simulink model "simulink_projekt3"  (R2023b)
settings: Solver=VariableStepAuto  StartTime=0.0  StopTime=5  RelTol=1e-3
settings Model: Creator=ingrj  LastModifiedBy=ingrj

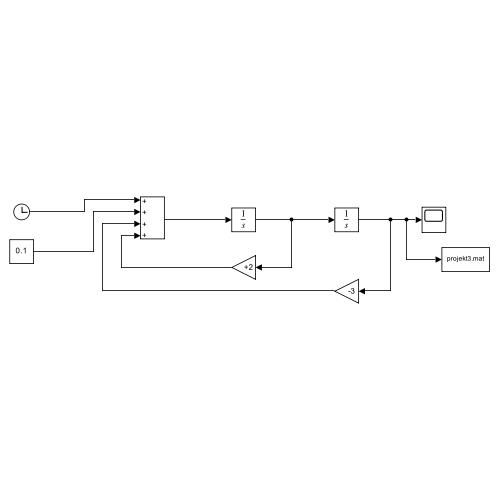
[thumbnail: Simulink's stored preview of the top-level diagram]
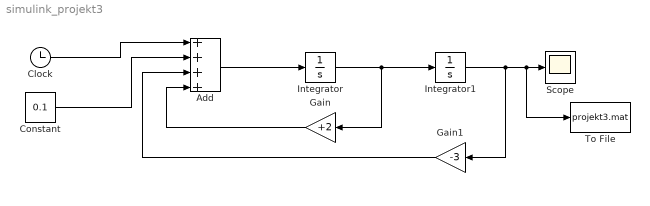
== system simulink_projekt3 ==
  Add : Sum  Inputs=++++
  Clock : Clock
  Constant : Constant  Value=0.1
  Gain : Gain  Gain=+2
  Gain1 : Gain  Gain=-3
  Integrator : Integrator  InitialCondition=1
  Integrator1 : Integrator
  Scope : Scope
  To File : ToFile  Filename=projekt3.mat  MatrixName=Sim  SaveFormat=Timeseries
  wires:
  Integrator/1 -> Gain/1, Integrator1/1
  Add/1 -> Integrator/1
  Gain/1 -> Add/4
  Integrator1/1 -> Gain1/1, To File/1, Scope/1
  Gain1/1 -> Add/3
  Clock/1 -> Add/1
  Constant/1 -> Add/2
